simulink model "battery"  (R2024b)
settings: Solver=VariableStepAuto  StartTime=0.0  StopTime=10.0  RelTol=1e-3
model workspace (MAT data in the model file):
  A_busbar = 0.0015
  A_pack = 0.711626248
  C_nominal = 3
  I_max = 157.708978328
  P = 5
  S = 138
  SoC_initial = 0.78
  T_amb = 297.15
  W_max = 34
  busbar_CC_area = 0.000108
  busbar_Cp = 237
  busbar_length = 0.032
  busbar_mass = 0.01
  busbar_resistivity = 1.68e-08
  busbar_thermalcontact_resistance = 1
  cell_Cp = 1000
  cell_mass = 0.046
  h_busbar = 5
  h_pack = 5
  pack_fuse = 175
settings Model: Creator=account  LastModifiedBy=account

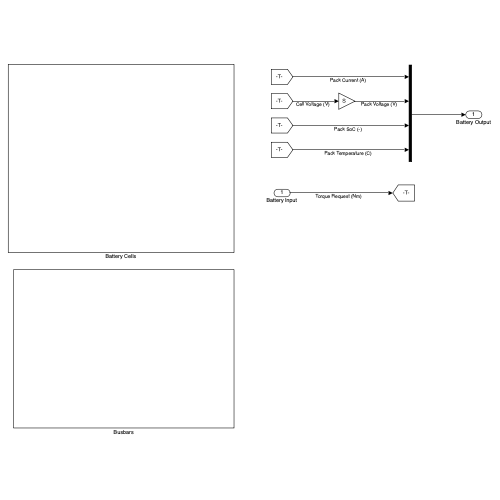
[thumbnail: Simulink's stored preview of the top-level diagram]
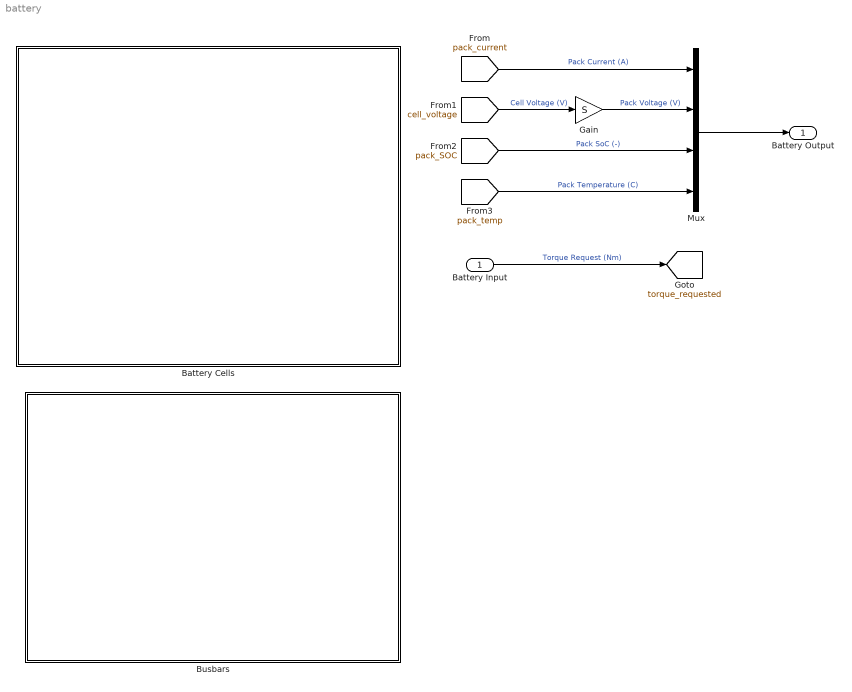
== system battery ==
  Battery Input : Inport
  Battery Cells : Subsystem
  Busbars : Subsystem
  Gain : Gain  Gain=S
  Mux : Mux
  Battery Output : Outport
  tag scope: torque_requested=global
  wires:
  [pack_SOC] -> Mux/3  "Pack SoC (-)"
  [pack_current] -> Mux/1  "Pack Current (A)"
  Gain/1 -> Mux/2  "Pack Voltage (V)"
  [pack_temp] -> Mux/4  "Pack Temperature (C)"
  [cell_voltage] -> Gain/1  "Cell Voltage (V)"
  Battery Input/1 -> [torque_requested]  "Torque Request (Nm)"
  Mux/1 -> Battery Output/1

== system battery/Battery Cells ==
  Battery Heat : Subsystem
      settings: PortSchema="{\"entries\":[{\"content\":{\"sides\":[{\"content\":{\"connectorIds\":[\"In1\",\"Out1\",\"In2\",\"In3\"]},\"type\":\"ConnectorPlacement.EquallySpacedRectSide\",\"uuid\":\"0f7c0562-63f7-413a-9c65-7d5d0f23ac53\"},{\"content\":{\"side\":\"RIGHT\"},\"type\":\"ConnectorPlacement.EquallySpacedRectSide\",\"uuid\":\"6856fc4a-e601-47fb-aafe-3183d6398fa2\"},{\"content\":{\"side\":\"TOP\"},\"type\":\"ConnectorPlacement.EquallySpacedRectSide\",\"uuid\":\"93500152-ab0c-4e86-a765-8796b82b9cd6\"}]},\"type\":\"ConnectorPlacement.EquallySpacedConnector\",\"uuid\":\"8bef09a8-0835-4033-ba4e-3f5f6277d0ac\"}],\"packageUris\":[\"http://schema.mathworks.com/mf0/Connector/R2020b\"],\"version\":\"1.0\"}"
  Battery Heat Generation : Subsystem
  Busbar - Segment Heat Flow : Subsystem
      settings: PortSchema="{\"entries\":[{\"content\":{\"sides\":[{\"content\":{},\"type\":\"ConnectorPlacement.EquallySpacedRectSide\",\"uuid\":\"839c7b7c-3d90-4543-803d-828e2cd8ee3e\"},{\"content\":{\"connectorIds\":[\"In1\",\"Out1\"],\"side\":\"RIGHT\"},\"type\":\"ConnectorPlacement.EquallySpacedRectSide\",\"uuid\":\"e3492608-3f40-473c-8392-0c925b682872\"},{\"content\":{\"side\":\"TOP\"},\"type\":\"ConnectorPlacement.EquallySpacedRectSide\",\"uuid\":\"8e15337c-e61d-491c-b508-620217c9bb60\"}]},\"type\":\"ConnectorPlacement.EquallySpacedConnector\",\"uuid\":\"03d3ec16-7a24-4203-9805-446eb586226e\"}],\"packageUris\":[\"http://schema.mathworks.com/mf0/Connector/R2020b\"],\"version\":\"1.0\"}"
  Heat Loss : Subsystem
      settings: PortSchema="{\"entries\":[{\"content\":{\"sides\":[{\"content\":{},\"type\":\"ConnectorPlacement.EquallySpacedRectSide\",\"uuid\":\"cd11f8f0-ebc0-4dda-8c98-00f5919de41a\"},{\"content\":{\"connectorIds\":[\"In1\",\"Out1\"],\"side\":\"RIGHT\"},\"type\":\"ConnectorPlacement.EquallySpacedRectSide\",\"uuid\":\"2a68a9a1-bd97-4a17-8a8b-1aa98e9bd9a8\"},{\"content\":{\"side\":\"TOP\"},\"type\":\"ConnectorPlacement.EquallySpacedRectSide\",\"uuid\":\"debcc510-941b-4448-a371-f67c84c59f32\"}]},\"type\":\"ConnectorPlacement.EquallySpacedConnector\",\"uuid\":\"91559e46-754b-48b4-ac3e-ab135f9add0a\"}],\"packageUris\":[\"http://schema.mathworks.com/mf0/Connector/R2020b\"],\"version\":\"1.0\"}"
  wires:
  Battery Heat/1(Pack Temp (K)) -> Busbar - Segment Heat Flow/1(Segment Temp (K)), Heat Loss/1(Pack Temp (K))
  Battery Heat Generation/1(Battery Heat Generation Rate) -> Battery Heat/1(Battery Heat Generation)
  Heat Loss/1(Pack Heat Loss Rate) -> Battery Heat/2(Battery Heat Loss)
  Busbar - Segment Heat Flow/1(Busbar - Segment Heat Flow (W)) -> Battery Heat/3(Busbar - Segment Heat Flow (W))

== system battery/Busbars ==
  Ambient Heat Loss : Subsystem
      settings: PortSchema="{\"entries\":[{\"content\":{\"sides\":[{\"content\":{},\"type\":\"ConnectorPlacement.EquallySpacedRectSide\",\"uuid\":\"cd11f8f0-ebc0-4dda-8c98-00f5919de41a\"},{\"content\":{\"connectorIds\":[\"In1\",\"Out1\"],\"side\":\"RIGHT\"},\"type\":\"ConnectorPlacement.EquallySpacedRectSide\",\"uuid\":\"2a68a9a1-bd97-4a17-8a8b-1aa98e9bd9a8\"},{\"content\":{\"side\":\"TOP\"},\"type\":\"ConnectorPlacement.EquallySpacedRectSide\",\"uuid\":\"debcc510-941b-4448-a371-f67c84c59f32\"}]},\"type\":\"ConnectorPlacement.EquallySpacedConnector\",\"uuid\":\"91559e46-754b-48b4-ac3e-ab135f9add0a\"}],\"packageUris\":[\"http://schema.mathworks.com/mf0/Connector/R2020b\"],\"version\":\"1.0\"}"
  Busbar - Segment Heat Flow : Subsystem
      settings: PortSchema="{\"entries\":[{\"content\":{\"sides\":[{\"content\":{},\"type\":\"ConnectorPlacement.EquallySpacedRectSide\",\"uuid\":\"839c7b7c-3d90-4543-803d-828e2cd8ee3e\"},{\"content\":{\"connectorIds\":[\"In1\",\"Out1\"],\"side\":\"RIGHT\"},\"type\":\"ConnectorPlacement.EquallySpacedRectSide\",\"uuid\":\"e3492608-3f40-473c-8392-0c925b682872\"},{\"content\":{\"side\":\"TOP\"},\"type\":\"ConnectorPlacement.EquallySpacedRectSide\",\"uuid\":\"8e15337c-e61d-491c-b508-620217c9bb60\"}]},\"type\":\"ConnectorPlacement.EquallySpacedConnector\",\"uuid\":\"03d3ec16-7a24-4203-9805-446eb586226e\"}],\"packageUris\":[\"http://schema.mathworks.com/mf0/Connector/R2020b\"],\"version\":\"1.0\"}"
  Busbar Heat : Subsystem
      settings: PortSchema="{\"entries\":[{\"content\":{\"sides\":[{\"content\":{\"connectorIds\":[\"In1\",\"Out1\",\"In2\",\"In3\"]},\"type\":\"ConnectorPlacement.EquallySpacedRectSide\",\"uuid\":\"0f7c0562-63f7-413a-9c65-7d5d0f23ac53\"},{\"content\":{\"side\":\"RIGHT\"},\"type\":\"ConnectorPlacement.EquallySpacedRectSide\",\"uuid\":\"6856fc4a-e601-47fb-aafe-3183d6398fa2\"},{\"content\":{\"side\":\"TOP\"},\"type\":\"ConnectorPlacement.EquallySpacedRectSide\",\"uuid\":\"93500152-ab0c-4e86-a765-8796b82b9cd6\"}]},\"type\":\"ConnectorPlacement.EquallySpacedConnector\",\"uuid\":\"8bef09a8-0835-4033-ba4e-3f5f6277d0ac\"}],\"packageUris\":[\"http://schema.mathworks.com/mf0/Connector/R2020b\"],\"version\":\"1.0\"}"
  Resistance Heat Generation : Subsystem
  wires:
  Busbar Heat/1(Busbar Temp (K)) -> Busbar - Segment Heat Flow/1(Busbar Temp (K)), Ambient Heat Loss/1(Busbar Temp (K))
  Resistance Heat Generation/1(Busbar Heat Generation Rate) -> Busbar Heat/1(Busbar Heat Generation)
  Ambient Heat Loss/1(Busbar Heat Loss Rate) -> Busbar Heat/2(Busbar Heat Loss)
  Busbar - Segment Heat Flow/1(Busbar - Segment Heat Flow (W)) -> Busbar Heat/3(Busbar - Segment Heat Flow (W))

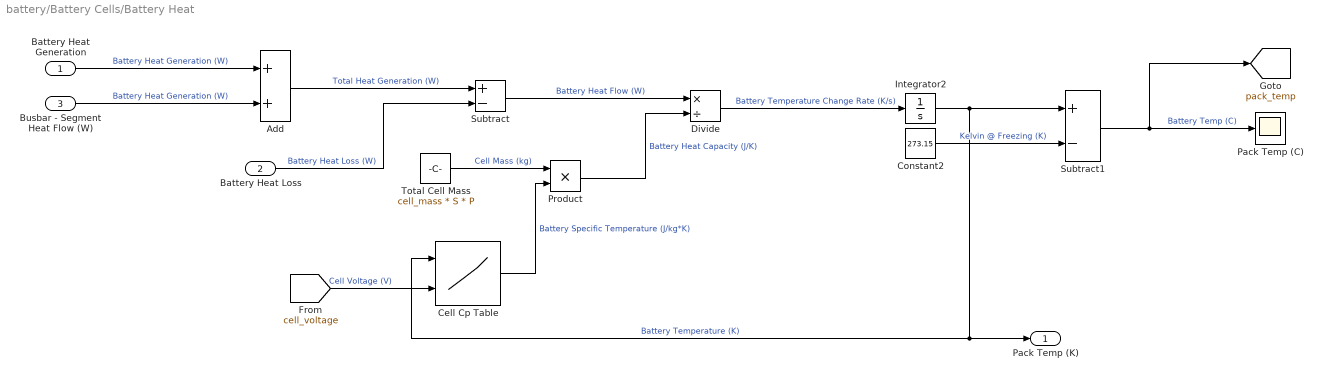
== system battery/Battery Cells/Battery Heat ==
  Battery Heat Generation : Inport
  Battery Heat Loss : Inport  Port=2
  Busbar - Segment Heat Flow (W) : Inport  Port=3
  Add : Sum
  Cell Cp Table : Lookup_n-D  BreakpointsForDimension1=[296.0488;303.3425;312.147;321.5769;330.6423]  BreakpointsForDimension2=[0 0.5 1]  Table=[811.0868 819.6535 830.8545;814.1373 822.704 834.6964;817.9826 826.8129 838.6737000000001;822.2249 831.0552 843.4446;826.7299 835.8239 848.3459]  InterpMethod=Cubic spline  InternalRulePriority=Speed  RndMeth=Simplest
      settings: InputPortMap=u0,u1
  Constant2 : Constant  Value=273.15
  Divide : Product  Inputs=*/
  Integrator2 : Integrator  InitialCondition=T_amb
  Pack Temp (C) : Scope
  Product : Product
  Subtract : Sum  Inputs=+-
  Subtract1 : Sum  Inputs=+-
  Total Cell Mass : Constant  Value=cell_mass * S * P
  Pack Temp (K) : Outport
  tag scope: pack_temp=global
  wires:
  Cell Cp Table/1 -> Product/2  "Battery Specific Temperature (J/kg*K)"
  Constant2/1 -> Subtract1/2  "Kelvin @ Freezing (K)"
  Divide/1 -> Integrator2/1  "Battery Temperature Change Rate (K/s)"
  Subtract/1 -> Divide/1  "Battery Heat Flow (W)"
  Integrator2/1 -> Cell Cp Table/1, Pack Temp (K)/1, Subtract1/1  "Battery Temperature (K)"
  Subtract1/1 -> [pack_temp], Pack Temp (C)/1  "Battery Temp (C)"
  Total Cell Mass/1 -> Product/1  "Cell Mass (kg)"
  Product/1 -> Divide/2  "Battery Heat Capacity (J/K)"
  Battery Heat Loss/1 -> Subtract/2  "Battery Heat Loss (W)"
  Battery Heat Generation/1 -> Add/1  "Battery Heat Generation (W)"
  Busbar - Segment Heat Flow (W)/1 -> Add/2  "Battery Heat Generation (W)"
  Add/1 -> Subtract/1  "Total Heat Generation (W)"
  [cell_voltage] -> Cell Cp Table/2  "Cell Voltage (V)"

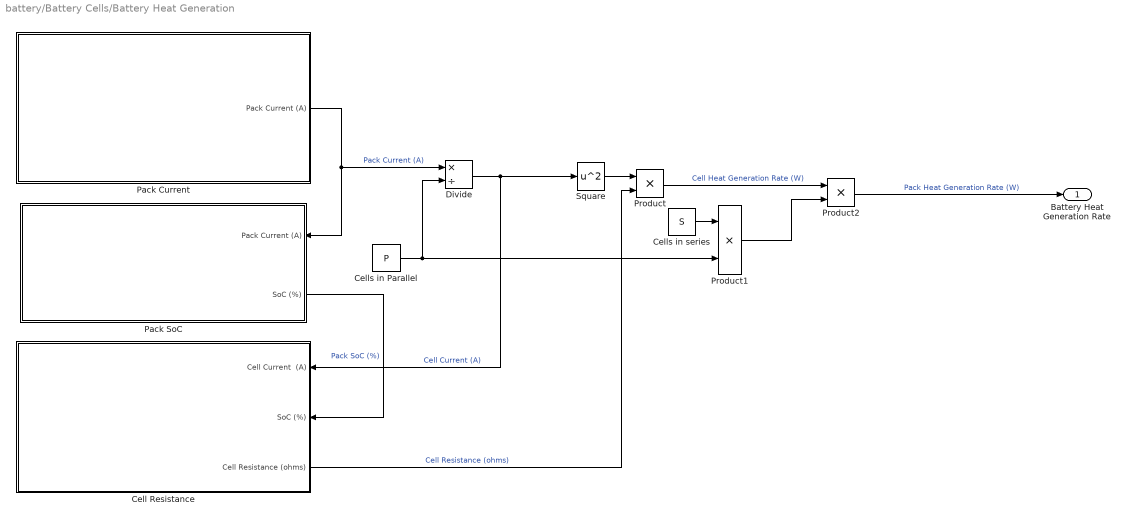
== system battery/Battery Cells/Battery Heat Generation ==
  Cell Resistance : Subsystem
      settings: PortSchema="{\"entries\":[{\"content\":{\"sides\":[{\"content\":{},\"type\":\"ConnectorPlacement.EquallySpacedRectSide\",\"uuid\":\"1c6ff2a8-2c86-4b92-aa7d-5717a02d6f28\"},{\"content\":{\"connectorIds\":[\"In1\",\"In2\",\"Out1\"],\"side\":\"RIGHT\"},\"type\":\"ConnectorPlacement.EquallySpacedRectSide\",\"uuid\":\"52a4cb2c-e1db-459d-bd0a-206cc3bba6d1\"},{\"content\":{\"side\":\"TOP\"},\"type\":\"ConnectorPlacement.EquallySpacedRectSide\",\"uuid\":\"751bbbd6-abc7-4265-8d68-4aa70d69379f\"}]},\"type\":\"ConnectorPlacement.EquallySpacedConnector\",\"uuid\":\"b8f9630f-0167-4478-8d98-637e13782dcd\"}],\"packageUris\":[\"http://schema.mathworks.com/mf0/Connector/R2020b\"],\"version\":\"1.0\"}"
      mask Display: image('resistor.png');
  Cells in Parallel : Constant  Value=P
  Cells in series : Constant  Value=S
  Divide : Product  Inputs=*/
  Pack Current : Subsystem
      mask Display: image('current.png');
  Pack SoC : Subsystem
      settings: PortSchema="{\"entries\":[{\"content\":{\"sides\":[{\"content\":{},\"type\":\"ConnectorPlacement.EquallySpacedRectSide\",\"uuid\":\"1c6ff2a8-2c86-4b92-aa7d-5717a02d6f28\"},{\"content\":{\"connectorIds\":[\"In1\",\"Out1\"],\"side\":\"RIGHT\"},\"type\":\"ConnectorPlacement.EquallySpacedRectSide\",\"uuid\":\"52a4cb2c-e1db-459d-bd0a-206cc3bba6d1\"},{\"content\":{\"side\":\"TOP\"},\"type\":\"ConnectorPlacement.EquallySpacedRectSide\",\"uuid\":\"751bbbd6-abc7-4265-8d68-4aa70d69379f\"}]},\"type\":\"ConnectorPlacement.EquallySpacedConnector\",\"uuid\":\"b8f9630f-0167-4478-8d98-637e13782dcd\"}],\"packageUris\":[\"http://schema.mathworks.com/mf0/Connector/R2020b\"],\"version\":\"1.0\"}"
      mask Display: image('SoC.jpg');
  Product : Product
  Product1 : Product
  Product2 : Product
  Square : Math  Operator=square
  Battery Heat Generation Rate : Outport
  wires:
  Cells in series/1 -> Product1/1
  Divide/1 -> Cell Resistance/1(Cell Current  (A)), Square/1  "Cell Current (A)"
  Cell Resistance/1(Cell Resistance (ohms)) -> Product/2  "Cell Resistance (ohms)"
  Square/1 -> Product/1
  Cells in Parallel/1 -> Divide/2, Product1/2
  Product1/1 -> Product2/2
  Product/1 -> Product2/1  "Cell Heat Generation Rate (W)"
  Product2/1 -> Battery Heat Generation Rate/1  "Pack Heat Generation Rate (W)"
  Pack SoC/1(SoC (%)) -> Cell Resistance/2(SoC (%))  "Pack SoC (%)"
  Pack Current/1(Pack Current (A)) -> Divide/1, Pack SoC/1(Pack Current (A))  "Pack Current (A)"

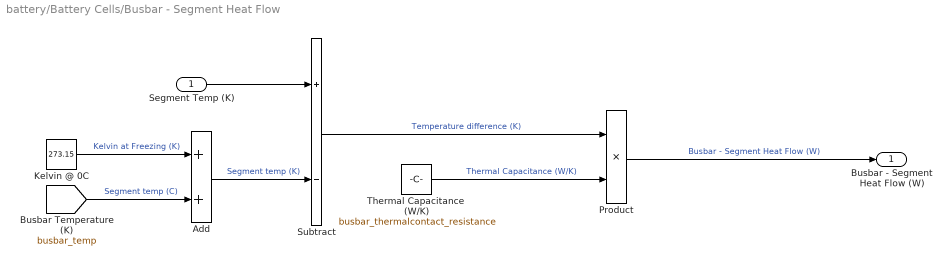
== system battery/Battery Cells/Busbar - Segment Heat Flow ==
  Segment Temp (K) : Inport
  Add : Sum
  Kelvin @ 0C : Constant  Value=273.15
  Product : Product
  Subtract : Sum  Inputs=+-
  Thermal Capacitance  (W/K) : Constant  Value=busbar_thermalcontact_resistance
  Busbar - Segment Heat Flow (W) : Outport
  wires:
  Subtract/1 -> Product/1  "Temperature difference (K)"
  Thermal Capacitance  (W/K)/1 -> Product/2  "Thermal Capacitance (W/K)"
  Product/1 -> Busbar - Segment Heat Flow (W)/1  "Busbar - Segment Heat Flow (W)"
  [busbar_temp] -> Add/2  "Segment temp (C)"
  Kelvin @ 0C/1 -> Add/1  "Kelvin at Freezing (K)"
  Segment Temp (K)/1 -> Subtract/1
  Add/1 -> Subtract/2  "Segment temp (K)"

== system battery/Battery Cells/Heat Loss ==
  Pack Temp (K) : Inport
  Ambient Temp (K) : Constant  Value=T_amb
  Pack Convective Heat Transfer Coefficient (W/m^2*K) : Constant  Value=h_pack
  Pack Surface Area (m^2) : Gain  Gain=A_pack
  Product : Product
  Subtract : Sum  Inputs=+-
  Pack Heat Loss Rate : Outport
  tag scope: pack_heatloss=global
  wires:
  Pack Convective Heat Transfer Coefficient (W/m^2*K)/1 -> Pack Surface Area (m^2)/1  "Pack Convective Heat Transfer Coefficient (W/m^2*K)"
  Subtract/1 -> Product/2  "Temperature Difference (K)"
  Pack Surface Area (m^2)/1 -> Product/1  "Heat Transfer Capacitance (W/K)"
  Product/1 -> [pack_heatloss], Pack Heat Loss Rate/1  "Pack Heat Loss Rate (W)"
  Pack Temp (K)/1 -> Subtract/1  "Pack Temp (K)"
  Ambient Temp (K)/1 -> Subtract/2  "Ambient Temp (K)"

== system battery/Busbars/Ambient Heat Loss ==
  Busbar Temp (K) : Inport
  Ambient temp (K) : Constant  Value=T_amb
  H busbar : Constant  Value=h_busbar
  Product : Product
  Subtract : Sum  Inputs=+-
  busbar area : Gain  Gain=A_busbar
  Busbar Heat Loss Rate : Outport
  tag scope: busbar_heatloss=global
  wires:
  H busbar/1 -> busbar area/1
  Subtract/1 -> Product/2
  busbar area/1 -> Product/1
  Product/1 -> [busbar_heatloss], Busbar Heat Loss Rate/1
  Busbar Temp (K)/1 -> Subtract/1
  Ambient temp (K)/1 -> Subtract/2

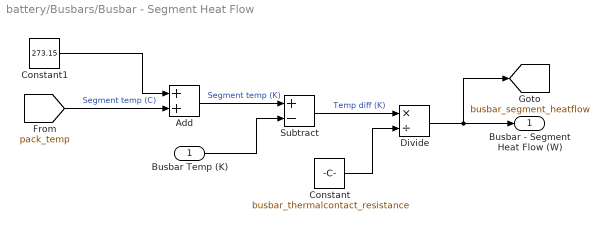
== system battery/Busbars/Busbar - Segment Heat Flow ==
  Busbar Temp (K) : Inport
  Add : Sum
  Constant : Constant  Value=busbar_thermalcontact_resistance
  Constant1 : Constant  Value=273.15
  Divide : Product  Inputs=*/
  Subtract : Sum  Inputs=+-
  Busbar - Segment Heat Flow (W) : Outport
  tag scope: busbar_segment_heatflow=global
  wires:
  Busbar Temp (K)/1 -> Subtract/2
  Subtract/1 -> Divide/1  "Temp diff (K)"
  Constant/1 -> Divide/2
  Divide/1 -> [busbar_segment_heatflow], Busbar - Segment Heat Flow (W)/1
  [pack_temp] -> Add/2  "Segment temp (C)"
  Constant1/1 -> Add/1
  Add/1 -> Subtract/1  "Segment temp (K)"

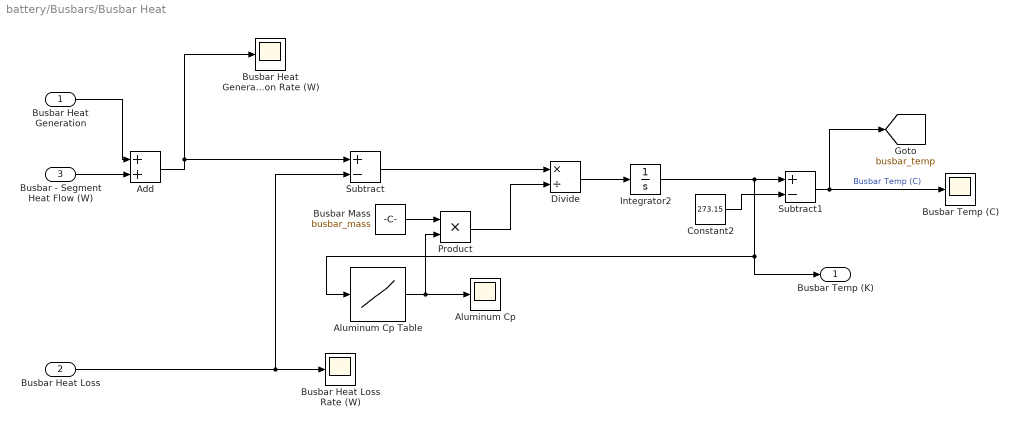
== system battery/Busbars/Busbar Heat ==
  Busbar Heat Generation : Inport
  Busbar Heat Loss : Inport  Port=2
  Busbar - Segment Heat Flow (W) : Inport  Port=3
  Add : Sum
  Aluminum Cp : Scope
  Aluminum Cp Table : Lookup_n-D  NumberOfTableDimensions=1  BreakpointsForDimension1=[298;300;400;500;600;700;800;900]  Table=[380.7;381.6;405.6;422.3;438.8;457.9;480.9;508.3]  InterpMethod=Cubic spline  InternalRulePriority=Speed  RndMeth=Simplest
  Busbar Heat Generation Rate (W) : Scope
  Busbar Heat Loss Rate (W) : Scope
  Busbar Mass : Constant  Value=busbar_mass
  Busbar Temp (C) : Scope
  Constant2 : Constant  Value=273.15
  Divide : Product  Inputs=*/
  Integrator2 : Integrator  InitialCondition=T_amb
  Product : Product
  Subtract : Sum  Inputs=+-
  Subtract1 : Sum  Inputs=+-
  Busbar Temp (K) : Outport
  tag scope: busbar_temp=global
  wires:
  Aluminum Cp Table/1 -> Product/2, Aluminum Cp/1
  Constant2/1 -> Subtract1/2
  Busbar Heat Generation/1 -> Add/1
  Divide/1 -> Integrator2/1
  Subtract/1 -> Divide/1
  Integrator2/1 -> Aluminum Cp Table/1, Busbar Temp (K)/1, Subtract1/1
  Subtract1/1 -> [busbar_temp], Busbar Temp (C)/1  "Busbar Temp (C)"
  Busbar Mass/1 -> Product/1
  Product/1 -> Divide/2
  Busbar Heat Loss/1 -> Busbar Heat Loss Rate (W)/1, Subtract/2
  Busbar - Segment Heat Flow (W)/1 -> Add/2
  Add/1 -> Subtract/1, Busbar Heat Generation Rate (W)/1

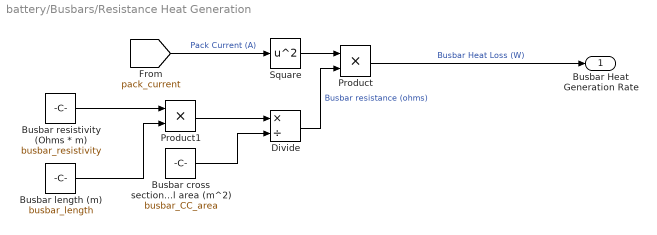
== system battery/Busbars/Resistance Heat Generation ==
  Busbar cross sectional area (m^2) : Constant  Value=busbar_CC_area
  Busbar length (m) : Constant  Value=busbar_length
  Busbar resistivity (Ohms * m) : Constant  Value=busbar_resistivity
  Divide : Product  Inputs=*/
  Product : Product
  Product1 : Product
  Square : Math  Operator=square
  Busbar Heat Generation Rate : Outport
  wires:
  Product/1 -> Busbar Heat Generation Rate/1  "Busbar Heat Loss (W)"
  [pack_current] -> Square/1  "Pack Current (A)"
  Square/1 -> Product/1
  Busbar resistivity (Ohms * m)/1 -> Product1/1
  Busbar length (m)/1 -> Product1/2
  Product1/1 -> Divide/1
  Busbar cross sectional area (m^2)/1 -> Divide/2
  Divide/1 -> Product/2  "Busbar resistance (ohms)"

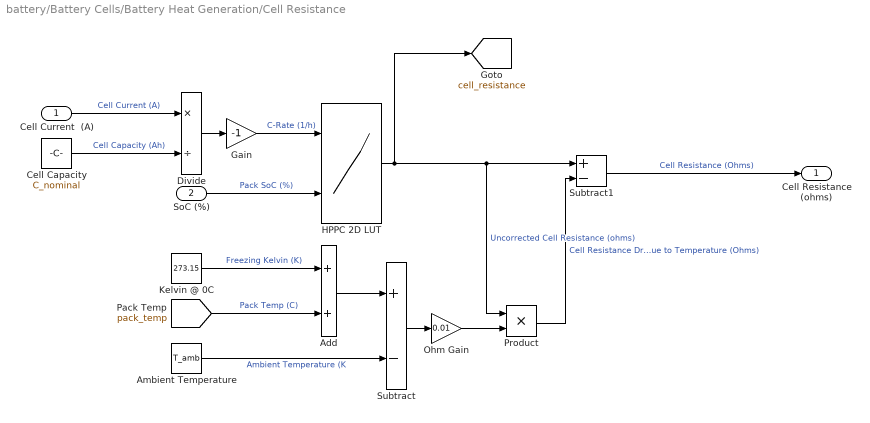
== system battery/Battery Cells/Battery Heat Generation/Cell Resistance ==
  Cell Current  (A) : Inport
  SoC (%) : Inport  Port=2
  Add : Sum
  Ambient Temperature : Constant  Value=T_amb
  Cell Capacity : Constant  Value=C_nominal
  Divide : Product  Inputs=*/
  Gain : Gain  Gain=-1
  HPPC 2D LUT : Lookup_n-D  BreakpointsForDimension1=[-10;-5;-1;1;2;3]  BreakpointsForDimension2=[0.1;0.2;0.3;0.4;0.5;0.6;0.7;0.8;0.9;1]  Table=[0.018906 0.01868 0.018453 0.018226 0.017999 0.017916 0.017743 0.018183 0.019549 0.022703;0.021356 0.020344 0.019332 0.019017 0.018694 0.018598 0.018319 0.018773 0.020642 0.024917;0.02305 0.020909 0.018859 0.019644 0.019687 0.018989 0.018291 0.019295 0.021608 0.026536;0.023001 0.020599 0.019683 0.019161 0.01894 0.018506 0.018636 0.019336 0.020993 0.02265;0.022654 0.020712 0.018901 0.018682 0.018442 0.018289 0.017788 0.017286 0.016785 0.016283;0.019898 0.017891 0.017366 0.01725 0.01725 0.017251 0.017251 0.017251 0.017251 0.017251]  InterpMethod=Cubic spline  ExtrapMethod=Clip  InternalRulePriority=Speed  RndMeth=Simplest
      settings: InputPortMap=u0,u1
  Kelvin @ 0C : Constant  Value=273.15
  Ohm Gain : Gain  Gain=0.01
  Product : Product
  Subtract : Sum  Inputs=+-
  Subtract1 : Sum  Inputs=+-
  Cell Resistance (ohms) : Outport
  tag scope: cell_resistance=global
  wires:
  Cell Current  (A)/1 -> Divide/1  "Cell Current (A)"
  Cell Capacity/1 -> Divide/2  "Cell Capacity (Ah)"
  SoC (%)/1 -> HPPC 2D LUT/2  "Pack SoC (%)"
  HPPC 2D LUT/1 -> [cell_resistance], Subtract1/1, Product/1  "Uncorrected Cell Resistance (ohms)"
  Divide/1 -> Gain/1
  Gain/1 -> HPPC 2D LUT/1  "C-Rate (1/h)"
  Subtract/1 -> Ohm Gain/1
  Ambient Temperature/1 -> Subtract/2  "Ambient Temperature (K"
  [pack_temp] -> Add/2  "Pack Temp (C)"
  Add/1 -> Subtract/1
  Kelvin @ 0C/1 -> Add/1  "Freezing Kelvin (K)"
  Ohm Gain/1 -> Product/2
  Product/1 -> Subtract1/2  "Cell Resistance Drop Due to Temperature (Ohms)"
  Subtract1/1 -> Cell Resistance (ohms)/1  "Cell Resistance (Ohms)"

== system battery/Battery Cells/Battery Heat Generation/Pack Current ==
  Divide : Product  Inputs=*/
  Fuse : Subsystem
  Gain : Gain  Gain=S
  Sony VTC6 Equivalent Circuit : Subsystem
  Pack Current (A) : Outport
  tag scope: pack_current=global
  wires:
  [torque_requested] -> Divide/1  "Driver Power Request (W)"
  Gain/1 -> Divide/2  "Pack Voltage (V)"
  Sony VTC6 Equivalent Circuit/1(Cell Voltage (V)) -> Gain/1  "Cell Voltage (V)"
  Divide/1 -> Fuse/1(Pack Current (A)), [pack_current], Pack Current (A)/1  "Pack Current (A)"

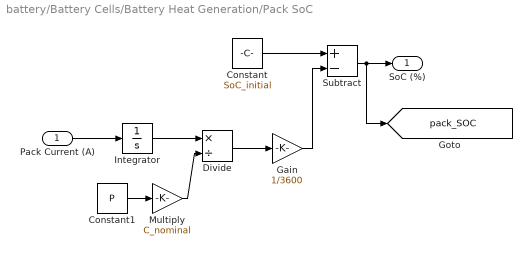
== system battery/Battery Cells/Battery Heat Generation/Pack SoC ==
  Pack Current (A) : Inport
  Constant : Constant  Value=SoC_initial
  Constant1 : Constant  Value=P
  Divide : Product  Inputs=*/
  Gain : Gain  Gain=1/3600
  Integrator : Integrator
  Multiply : Gain  Gain=C_nominal
  Subtract : Sum  Inputs=+-
  SoC (%) : Outport
  tag scope: pack_SOC=global
  wires:
  Pack Current (A)/1 -> Integrator/1
  Constant/1 -> Subtract/1
  Integrator/1 -> Divide/1
  Subtract/1 -> [pack_SOC], SoC (%)/1
  Constant1/1 -> Multiply/1
  Multiply/1 -> Divide/2
  Divide/1 -> Gain/1
  Gain/1 -> Subtract/2

== system battery/Battery Cells/Battery Heat Generation/Pack Current/Fuse ==
  Pack Current (A) : Inport
  Constant : Constant
  Constant1 : Constant  Value=0
  Stop Simulation : Stop
  Switch : Switch  Criteria=u2 > Threshold  Threshold=pack_fuse  SaturateOnIntegerOverflow=off  InputSameDT=off
  wires:
  Switch/1 -> Stop Simulation/1
  Pack Current (A)/1 -> Switch/2
  Constant/1 -> Switch/1
  Constant1/1 -> Switch/3

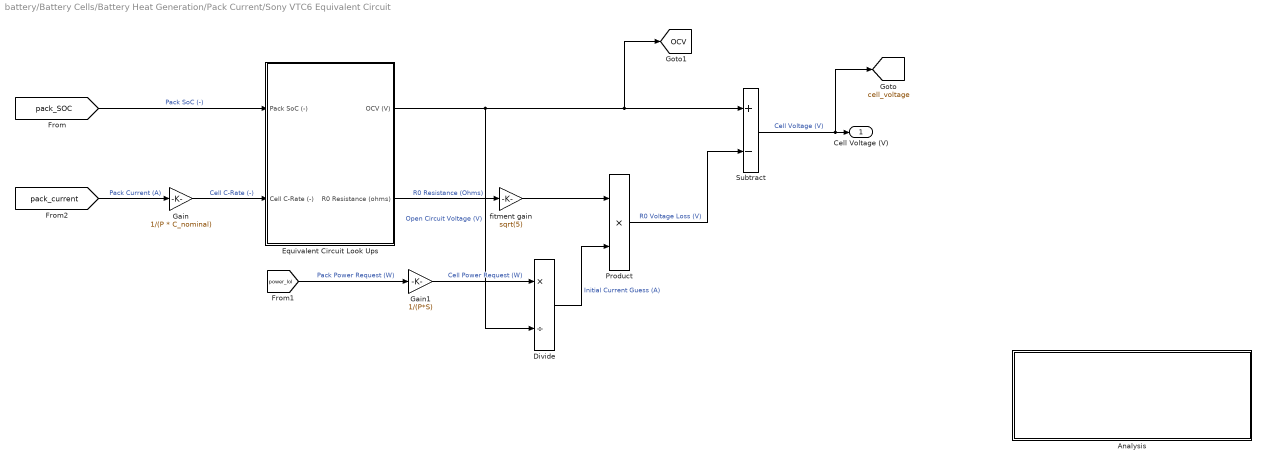
== system battery/Battery Cells/Battery Heat Generation/Pack Current/Sony VTC6 Equivalent Circuit ==
  Analysis : Subsystem
  Divide : Product  Inputs=*/
  Equivalent Circuit Look Ups : Subsystem
  Gain : Gain  Gain=1/(P * C_nominal)
  Gain1 : Gain  Gain=1/(P*S)
  Product : Product
  Subtract : Sum  Inputs=+-
  fitment gain : Gain  Gain=sqrt(5)
  Cell Voltage (V) : Outport
  tag scope: OCV=global, cell_voltage=global
  wires:
  [pack_SOC] -> Equivalent Circuit Look Ups/1(Pack SoC (-))  "Pack SoC (-)"
  Gain/1 -> Equivalent Circuit Look Ups/2(Cell C-Rate (-))  "Cell C-Rate (-)"
  Equivalent Circuit Look Ups/2(R0 Resistance (ohms)) -> fitment gain/1  "R0 Resistance (Ohms)"
  Equivalent Circuit Look Ups/1(OCV (V)) -> [OCV], Subtract/1, Divide/2  "Open Circuit Voltage (V)"
  Product/1 -> Subtract/2  "R0 Voltage Loss (V)"
  Subtract/1 -> [cell_voltage], Cell Voltage (V)/1  "Cell Voltage (V)"
  Divide/1 -> Product/2  "Initial Current Guess (A)"
  [power_lol] -> Gain1/1  "Pack Power Request (W)"
  Gain1/1 -> Divide/1  "Cell Power Request (W)"
  [pack_current] -> Gain/1  "Pack Current (A)"
  fitment gain/1 -> Product/1

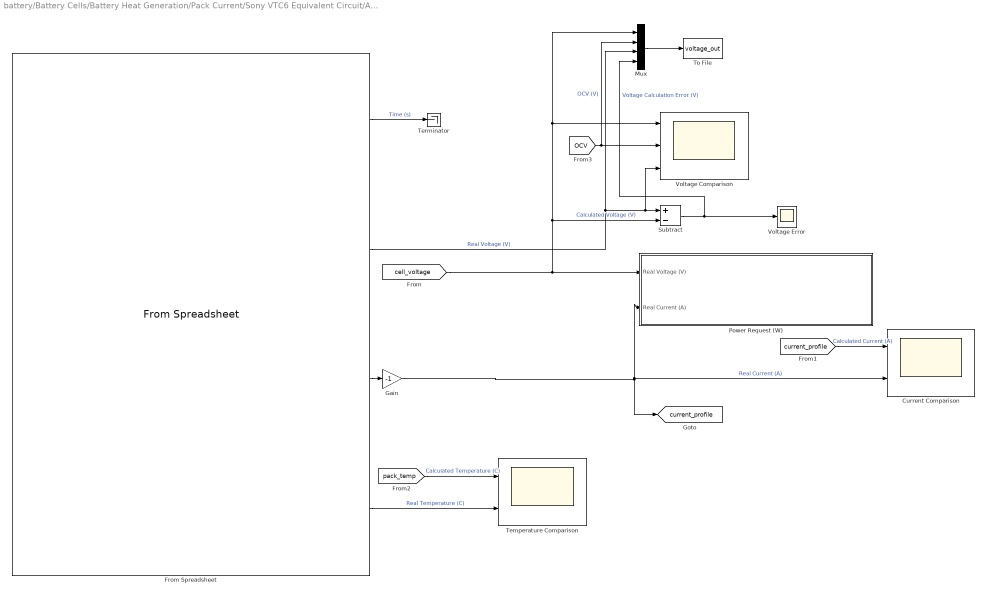
== system battery/Battery Cells/Battery Heat Generation/Pack Current/Sony VTC6 Equivalent Circuit/Analysis ==
  Current Comparison : Scope  NumInputPorts=2
  From Spreadsheet : FromSpreadsheet  FileName=arbincomparisondata.xlsx  TreatFirstColumnAs=Data  SampleTime=0.003
  Gain : Gain  Gain=-1
  Mux : Mux
  Power Request (W) : Subsystem
  Subtract : Sum  Inputs=+-
  Temperature Comparison : Scope  NumInputPorts=2
  Terminator : Terminator
  To File : ToFile  Filename=voltage_out  MatrixName=voltage  SampleTime=0.01
  Voltage Comparison : Scope  NumInputPorts=3
  Voltage Error : Scope
  tag scope: current_profile=global
  wires:
  [cell_voltage] -> Power Request (W)/1(Real Voltage (V)), Subtract/2, Mux/1, Voltage Comparison/1  "Calculated Voltage (V)"
  [current_profile] -> Current Comparison/1  "Calculated Current (A)"
  [pack_temp] -> Temperature Comparison/1  "Calculated Temperature (C)"
  From Spreadsheet/2 -> Mux/3, Subtract/1, Voltage Comparison/3  "Real Voltage (V)"
  From Spreadsheet/3 -> Gain/1
  From Spreadsheet/4 -> Temperature Comparison/2  "Real Temperature (C)"
  From Spreadsheet/1 -> Terminator/1  "Time (s)"
  Gain/1 -> Current Comparison/2, Power Request (W)/2(Real Current (A)), [current_profile]  "Real Current (A)"
  Subtract/1 -> Mux/4, Voltage Error/1  "Voltage Calculation Error (V)"
  [OCV] -> Mux/2, Voltage Comparison/2  "OCV (V)"
  Mux/1 -> To File/1

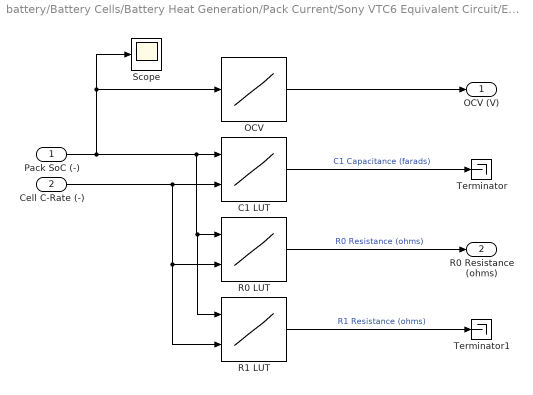
== system battery/Battery Cells/Battery Heat Generation/Pack Current/Sony VTC6 Equivalent Circuit/Equivalent Circuit Look Ups ==
  Pack SoC (-) : Inport
  Cell C-Rate (-) : Inport  Port=2
  C1 LUT : Lookup_n-D  BreakpointsForDimension1=[0.1;0.2;0.3;0.4;0.5;0.6;0.7;0.8;0.9;1]  BreakpointsForDimension2=[-10;-5;-1;-0.333;0.333;1;2;3]  Table=[0.018906 0.021356 0.02305 0.022911 0.023301 0.023001 0.022654 0.019898;0.01868 0.020344 0.020909 0.020815 0.020944 0.020599 0.020712 0.017891;0.018453 0.019332 0.018859 0.023564 0.020028 0.019683 0.018901 0.017366;0.018226 0.019017 0.019644 0.020423 0.019635 0.019161 0.018682 0.01725;0.017999 0.018694 0.019687 0.020161 0.019897 0.01894 0.018442 0.01725;0.017916 0.018598 0.018989 0.01859 0.019505 0.018506 0.018289 0.017251;0.017743 0.018319 0.018291 0.022256 0.019767 0.018636 0.017788 0.017251;0.018183 0.018773 0.019295 0.021996 0.019898 0.019336 0.017286 0.017251;0.019549 0.020642 0.021608 0.025136 0.022253 0.020993 0.016785 0.017251;0.022703 0.024917 0.026536 0.026706 0.024609 0.02265 0.016283 0.017251]  ExtrapMethod=Clip  InternalRulePriority=Speed  RndMeth=Simplest
      settings: InputPortMap=u0,u1
  OCV : Lookup_n-D  NumberOfTableDimensions=1  BreakpointsForDimension1=[0.1;0.2;0.3;0.4;0.5;0.6;0.7;0.8;0.9;1]  BeginIndexSearchUsingPreviousIndexResult=on  Table=[3.227877;3.437376;3.537935;3.663634;3.755814;3.835423;3.940172;4.047017;4.097296;4.187904]  InternalRulePriority=Speed  RndMeth=Simplest
  R0 LUT : Lookup_n-D  BreakpointsForDimension1=[0.1;0.2;0.3;0.4;0.5;0.6;0.7;0.8;0.9;1]  BreakpointsForDimension2=[-10;-5;-1;-0.333;0.333;1;2;3]  Table=[0.018906 0.021356 0.02305 0.022911 0.023301 0.023001 0.022654 0.019898;0.01868 0.020344 0.020909 0.020815 0.020944 0.020599 0.020712 0.017891;0.018453 0.019332 0.018859 0.023564 0.020028 0.019683 0.018901 0.017366;0.018226 0.019017 0.019644 0.020423 0.019635 0.019161 0.018682 0.01725;0.017999 0.018694 0.019687 0.020161 0.019897 0.01894 0.018442 0.01725;0.017916 0.018598 0.018989 0.01859 0.019505 0.018506 0.018289 0.017251;0.017743 0.018319 0.018291 0.022256 0.019767 0.018636 0.017788 0.017251;0.018183 0.018773 0.019295 0.021996 0.019898 0.019336 0.017286 0.017251;0.019549 0.020642 0.021608 0.025136 0.022253 0.020993 0.016785 0.017251;0.022703 0.024917 0.026536 0.026706 0.024609 0.02265 0.016283 0.017251]  ExtrapMethod=Clip  InternalRulePriority=Speed  RndMeth=Simplest
      settings: InputPortMap=u0,u1
  R1 LUT : Lookup_n-D  BreakpointsForDimension1=[0.1;0.2;0.3;0.4;0.5;0.6;0.7;0.8;0.9;1]  BreakpointsForDimension2=[-10;-5;-1;-0.333;0.333;1;2;3]  Table=[0.018906 0.021356 0.02305 0.022911 0.023301 0.023001 0.022654 0.019898;0.01868 0.020344 0.020909 0.020815 0.020944 0.020599 0.020712 0.017891;0.018453 0.019332 0.018859 0.023564 0.020028 0.019683 0.018901 0.017366;0.018226 0.019017 0.019644 0.020423 0.019635 0.019161 0.018682 0.01725;0.017999 0.018694 0.019687 0.020161 0.019897 0.01894 0.018442 0.01725;0.017916 0.018598 0.018989 0.01859 0.019505 0.018506 0.018289 0.017251;0.017743 0.018319 0.018291 0.022256 0.019767 0.018636 0.017788 0.017251;0.018183 0.018773 0.019295 0.021996 0.019898 0.019336 0.017286 0.017251;0.019549 0.020642 0.021608 0.025136 0.022253 0.020993 0.016785 0.017251;0.022703 0.024917 0.026536 0.026706 0.024609 0.02265 0.016283 0.017251]  InternalRulePriority=Speed  RndMeth=Simplest
      settings: InputPortMap=u0,u1
  Scope : Scope
  Terminator : Terminator
  Terminator1 : Terminator
  OCV (V) : Outport
  R0 Resistance (ohms) : Outport  Port=2
  wires:
  Cell C-Rate (-)/1 -> R1 LUT/2, R0 LUT/2, C1 LUT/2
  Pack SoC (-)/1 -> Scope/1, OCV/1, C1 LUT/1, R1 LUT/1, R0 LUT/1
  C1 LUT/1 -> Terminator/1  "C1 Capacitance (farads)"
  R1 LUT/1 -> Terminator1/1  "R1 Resistance (ohms)"
  R0 LUT/1 -> R0 Resistance (ohms)/1  "R0 Resistance (ohms)"
  OCV/1 -> OCV (V)/1

== system battery/Battery Cells/Battery Heat Generation/Pack Current/Sony VTC6 Equivalent Circuit/Analysis/Power Request (W) ==
  Real Voltage (V) : Inport
  Real Current (A) : Inport  Port=2
  Gain : Gain  Gain=S
  Product : Product
  tag scope: power_lol=global
  wires:
  Real Voltage (V)/1 -> Gain/1
  Gain/1 -> Product/1
  Real Current (A)/1 -> Product/2
  Product/1 -> [power_lol]
